simulink model "Distribution"  (R2015b)
settings: Solver=ode45  SolverMode=SingleTasking  StartTime=0.0  StopTime=500  RelTol=1e-3
libraries: simeventslib x10
(part 1 of 2)
settings Model: Creator=tsprock3  LastModifiedBy=tsprock3
settings DataIOCC: SaveFormat=Array
settings OptimizationCC: BlockReduction=off  BooleanDataType=off
settings DebuggingCC: SaveWithParameterizedLinksMsg=none  UnderspecifiedInitializationDetection=Classic  MergeDetectMultiDrivingBlocksExec=none  SignalResolutionControl=TryResolveAllWithWarning
settings HardwareCC: ProdBitPerPointer=32  ProdLargestAtomicFloat=None  ProdIntDivRoundTo=Undefined  ProdEndianess=Unspecified  ProdWordSize=32  ProdHWDeviceType=32-bit Generic  TargetUnknown=on
settings GRTTargetCC: GeneratePreprocessorConditionals=Disable all
settings ConfigComp: CovModelRefEnable=Off
settings SimEventsCC: propMaxDesBlkSimulEvents=100000  propMaxDesMdlSimulEvents=1000000

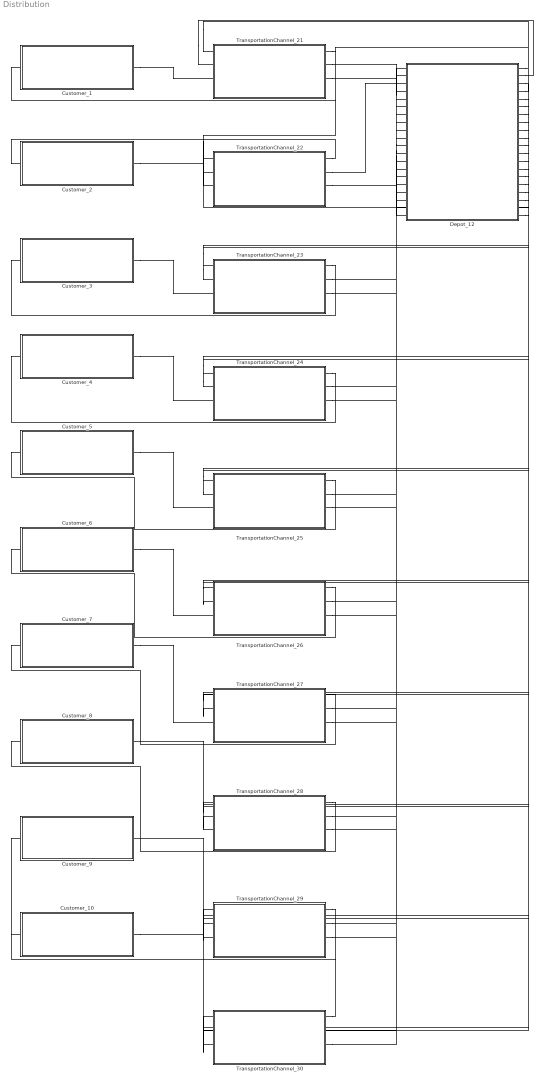
== system Distribution ==
  Customer_1 : Subsystem
  Customer_10 : Subsystem
  Customer_2 : Subsystem
  Customer_3 : Subsystem
  Customer_4 : Subsystem
  Customer_5 : Subsystem
  Customer_6 : Subsystem
  Customer_7 : Subsystem
  Customer_8 : Subsystem
  Customer_9 : Subsystem
  Depot_12 : Subsystem
  TransportationChannel_21 : Subsystem
  TransportationChannel_22 : Subsystem
  TransportationChannel_23 : Subsystem
  TransportationChannel_24 : Subsystem
  TransportationChannel_25 : Subsystem
  TransportationChannel_26 : Subsystem
  TransportationChannel_27 : Subsystem
  TransportationChannel_28 : Subsystem
  TransportationChannel_29 : Subsystem
  TransportationChannel_30 : Subsystem
  connections:
  Depot_12/RConn1 -- TransportationChannel_21/LConn1
  TransportationChannel_21/RConn1 -- Customer_1/LConn1
  Depot_12/RConn2 -- TransportationChannel_21/LConn2
  TransportationChannel_21/RConn2 -- Depot_12/LConn1
  Customer_1/RConn1 -- TransportationChannel_21/LConn3
  TransportationChannel_21/RConn3 -- Depot_12/LConn2
  Depot_12/RConn3 -- TransportationChannel_22/LConn1
  TransportationChannel_22/RConn1 -- Customer_2/LConn1
  Depot_12/RConn4 -- TransportationChannel_22/LConn2
  TransportationChannel_22/RConn2 -- Depot_12/LConn3
  Customer_2/RConn1 -- TransportationChannel_22/LConn3
  TransportationChannel_22/RConn3 -- Depot_12/LConn4
  Depot_12/RConn5 -- TransportationChannel_23/LConn1
  TransportationChannel_23/RConn1 -- Customer_3/LConn1
  Depot_12/RConn6 -- TransportationChannel_23/LConn2
  TransportationChannel_23/RConn2 -- Depot_12/LConn5
  Customer_3/RConn1 -- TransportationChannel_23/LConn3
  TransportationChannel_23/RConn3 -- Depot_12/LConn6
  Depot_12/RConn7 -- TransportationChannel_24/LConn1
  TransportationChannel_24/RConn1 -- Customer_4/LConn1
  Depot_12/RConn8 -- TransportationChannel_24/LConn2
  TransportationChannel_24/RConn2 -- Depot_12/LConn7
  Customer_4/RConn1 -- TransportationChannel_24/LConn3
  TransportationChannel_24/RConn3 -- Depot_12/LConn8
  Depot_12/RConn9 -- TransportationChannel_25/LConn1
  TransportationChannel_25/RConn1 -- Customer_5/LConn1
  Depot_12/RConn10 -- TransportationChannel_25/LConn2
  TransportationChannel_25/RConn2 -- Depot_12/LConn9
  Customer_5/RConn1 -- TransportationChannel_25/LConn3
  TransportationChannel_25/RConn3 -- Depot_12/LConn10
  Depot_12/RConn11 -- TransportationChannel_26/LConn1
  TransportationChannel_26/RConn1 -- Customer_6/LConn1
  Depot_12/RConn12 -- TransportationChannel_26/LConn2
  TransportationChannel_26/RConn2 -- Depot_12/LConn11
  Customer_6/RConn1 -- TransportationChannel_26/LConn3
  TransportationChannel_26/RConn3 -- Depot_12/LConn12
  Depot_12/RConn13 -- TransportationChannel_27/LConn1
  TransportationChannel_27/RConn1 -- Customer_7/LConn1
  Depot_12/RConn14 -- TransportationChannel_27/LConn2
  TransportationChannel_27/RConn2 -- Depot_12/LConn13
  Customer_7/RConn1 -- TransportationChannel_27/LConn3
  TransportationChannel_27/RConn3 -- Depot_12/LConn14
  Depot_12/RConn15 -- TransportationChannel_28/LConn1
  TransportationChannel_28/RConn1 -- Customer_8/LConn1
  Depot_12/RConn16 -- TransportationChannel_28/LConn2
  TransportationChannel_28/RConn2 -- Depot_12/LConn15
  Customer_8/RConn1 -- TransportationChannel_28/LConn3
  TransportationChannel_28/RConn3 -- Depot_12/LConn16
  Depot_12/RConn17 -- TransportationChannel_29/LConn1
  TransportationChannel_29/RConn1 -- Customer_9/LConn1
  Depot_12/RConn18 -- TransportationChannel_29/LConn2
  TransportationChannel_29/RConn2 -- Depot_12/LConn17
  Customer_9/RConn1 -- TransportationChannel_29/LConn3
  TransportationChannel_29/RConn3 -- Depot_12/LConn18
  Depot_12/RConn19 -- TransportationChannel_30/LConn1
  TransportationChannel_30/RConn1 -- Customer_10/LConn1
  Depot_12/RConn20 -- TransportationChannel_30/LConn2
  TransportationChannel_30/RConn2 -- Depot_12/LConn19
  Customer_10/RConn1 -- TransportationChannel_30/LConn3
  TransportationChannel_30/RConn3 -- Depot_12/LConn20

== system Distribution/Customer_1 ==
  Commodity_1 : Subsystem  mask{Mean=2000/2134, AttributeValue=[0]|1|0|1}
      mask prompts: Mean "Frequency"; AttributeValue "Attributes"
      mask TypeOptions Mean: Source/Mean
      mask TypeOptions AttributeValue: setAttribute/AttributeValue
  Entity Sink : EntitySink
  Get Attribute : GetAttribute  AttributeName=Origin|Destination|Start  AttributeMissing=Error|Error|Error  AttributeDefaultValue=1|1|1  AttributeTreatAsVector=1|1|1  AttributeSendTiming=After entity departure|After entity departure|After entity departure  EvaluatedDefaultAttributeValue={[];[];[]}
      settings: OutputPortMap=o1,o2,o3
  IN_Commodity : PathCombiner  NumberInputPorts=1
  IN_Shipment : PathCombiner  NumberInputPorts=1
  Mux : Mux  Inputs=3
  OUT_Shipment : OutputSwitch  NumberOutputPorts=1  SwitchingCriterion=From signal port p  AttributeName=Customer  StatNumberDeparted=on
  Routing : EventBasedRandomNumber  Distribution=Arbitrary discrete  valueVecDisc=[0,1]  probVecDisc=[0,1]  Seed=56944
  Shipment_Metrics : simeventslib/SimEvents Sinks/Discrete Event Signal to Workspace  VariableName=Customer_1  SaveFormat=Structure With Time  isMonitorOnly=off  isRecordIC=off
  Signal Latch : SignalLatch  InitialMemoryValue=1  ReadMemoryUpon=Write to memory event
      settings: InputPortMap=u0,u2  OutputPortMap=o2
  IN_Shipment_1 : PMIOPort  Port=1  Side=Left
  OUT_Shipment_1 : PMIOPort  Port=2  Side=Right
  wires:
  Signal Latch/1 -> OUT_Shipment/1
  OUT_Shipment/1 -> Signal Latch/1
  Routing/1 -> Signal Latch/2
  Mux/1 -> Shipment_Metrics/1
  Get Attribute/3 -> Mux/3
  Get Attribute/2 -> Mux/2
  Get Attribute/1 -> Mux/1
  connections:
  IN_Commodity/RConn1 -- OUT_Shipment/LConn1
  Get Attribute/LConn1 -- IN_Shipment/RConn1
  Entity Sink/LConn1 -- Get Attribute/RConn1
  IN_Shipment/LConn1 -- IN_Shipment_1/RConn1
  OUT_Shipment/RConn1 -- OUT_Shipment_1/RConn1
  Commodity_1/RConn1 -- IN_Commodity/LConn1

== system Distribution/Customer_10 ==
  Commodity_10 : Subsystem  mask{Mean=2000/1539, AttributeValue=[0]|10|0|1}
      mask prompts: Mean "Frequency"; AttributeValue "Attributes"
      mask TypeOptions Mean: Source/Mean
      mask TypeOptions AttributeValue: setAttribute/AttributeValue
  Entity Sink : EntitySink
  Get Attribute : GetAttribute  AttributeName=Origin|Destination|Start  AttributeMissing=Error|Error|Error  AttributeDefaultValue=1|1|1  AttributeTreatAsVector=1|1|1  AttributeSendTiming=After entity departure|After entity departure|After entity departure  EvaluatedDefaultAttributeValue={[];[];[]}
      settings: OutputPortMap=o1,o2,o3
  IN_Commodity : PathCombiner  NumberInputPorts=1
  IN_Shipment : PathCombiner  NumberInputPorts=1
  Mux : Mux  Inputs=3
  OUT_Shipment : OutputSwitch  NumberOutputPorts=1  SwitchingCriterion=From signal port p  AttributeName=Customer  StatNumberDeparted=on
  Routing : EventBasedRandomNumber  Distribution=Arbitrary discrete  valueVecDisc=[0,1]  probVecDisc=[0,1]  Seed=60161
  Shipment_Metrics : simeventslib/SimEvents Sinks/Discrete Event Signal to Workspace  VariableName=Customer_10  SaveFormat=Structure With Time  isMonitorOnly=off  isRecordIC=off
  Signal Latch : SignalLatch  InitialMemoryValue=1  ReadMemoryUpon=Write to memory event
      settings: InputPortMap=u0,u2  OutputPortMap=o2
  IN_Shipment_1 : PMIOPort  Port=1  Side=Left
  OUT_Shipment_1 : PMIOPort  Port=2  Side=Right
  wires:
  Signal Latch/1 -> OUT_Shipment/1
  OUT_Shipment/1 -> Signal Latch/1
  Routing/1 -> Signal Latch/2
  Mux/1 -> Shipment_Metrics/1
  Get Attribute/3 -> Mux/3
  Get Attribute/2 -> Mux/2
  Get Attribute/1 -> Mux/1
  connections:
  IN_Commodity/RConn1 -- OUT_Shipment/LConn1
  Get Attribute/LConn1 -- IN_Shipment/RConn1
  Entity Sink/LConn1 -- Get Attribute/RConn1
  IN_Shipment/LConn1 -- IN_Shipment_1/RConn1
  OUT_Shipment/RConn1 -- OUT_Shipment_1/RConn1
  Commodity_10/RConn1 -- IN_Commodity/LConn1

== system Distribution/Customer_2 ==
  Commodity_2 : Subsystem  mask{Mean=2000/1918, AttributeValue=[0]|2|0|1}
      mask prompts: Mean "Frequency"; AttributeValue "Attributes"
      mask TypeOptions Mean: Source/Mean
      mask TypeOptions AttributeValue: setAttribute/AttributeValue
  Entity Sink : EntitySink
  Get Attribute : GetAttribute  AttributeName=Origin|Destination|Start  AttributeMissing=Error|Error|Error  AttributeDefaultValue=1|1|1  AttributeTreatAsVector=1|1|1  AttributeSendTiming=After entity departure|After entity departure|After entity departure  EvaluatedDefaultAttributeValue={[];[];[]}
      settings: OutputPortMap=o1,o2,o3
  IN_Commodity : PathCombiner  NumberInputPorts=1
  IN_Shipment : PathCombiner  NumberInputPorts=1
  Mux : Mux  Inputs=3
  OUT_Shipment : OutputSwitch  NumberOutputPorts=1  SwitchingCriterion=From signal port p  AttributeName=Customer  StatNumberDeparted=on
  Routing : EventBasedRandomNumber  Distribution=Arbitrary discrete  valueVecDisc=[0,1]  probVecDisc=[0,1]  Seed=63378
  Shipment_Metrics : simeventslib/SimEvents Sinks/Discrete Event Signal to Workspace  VariableName=Customer_2  SaveFormat=Structure With Time  isMonitorOnly=off  isRecordIC=off
  Signal Latch : SignalLatch  InitialMemoryValue=1  ReadMemoryUpon=Write to memory event
      settings: InputPortMap=u0,u2  OutputPortMap=o2
  IN_Shipment_1 : PMIOPort  Port=1  Side=Left
  OUT_Shipment_1 : PMIOPort  Port=2  Side=Right
  wires:
  Signal Latch/1 -> OUT_Shipment/1
  OUT_Shipment/1 -> Signal Latch/1
  Routing/1 -> Signal Latch/2
  Mux/1 -> Shipment_Metrics/1
  Get Attribute/3 -> Mux/3
  Get Attribute/2 -> Mux/2
  Get Attribute/1 -> Mux/1
  connections:
  IN_Commodity/RConn1 -- OUT_Shipment/LConn1
  Get Attribute/LConn1 -- IN_Shipment/RConn1
  Entity Sink/LConn1 -- Get Attribute/RConn1
  IN_Shipment/LConn1 -- IN_Shipment_1/RConn1
  OUT_Shipment/RConn1 -- OUT_Shipment_1/RConn1
  Commodity_2/RConn1 -- IN_Commodity/LConn1

== system Distribution/Customer_3 ==
  Commodity_3 : Subsystem  mask{Mean=2000/1442, AttributeValue=[0]|3|0|1}
      mask prompts: Mean "Frequency"; AttributeValue "Attributes"
      mask TypeOptions Mean: Source/Mean
      mask TypeOptions AttributeValue: setAttribute/AttributeValue
  Entity Sink : EntitySink
  Get Attribute : GetAttribute  AttributeName=Origin|Destination|Start  AttributeMissing=Error|Error|Error  AttributeDefaultValue=1|1|1  AttributeTreatAsVector=1|1|1  AttributeSendTiming=After entity departure|After entity departure|After entity departure  EvaluatedDefaultAttributeValue={[];[];[]}
      settings: OutputPortMap=o1,o2,o3
  IN_Commodity : PathCombiner  NumberInputPorts=1
  IN_Shipment : PathCombiner  NumberInputPorts=1
  Mux : Mux  Inputs=3
  OUT_Shipment : OutputSwitch  NumberOutputPorts=1  SwitchingCriterion=From signal port p  AttributeName=Customer  StatNumberDeparted=on
  Routing : EventBasedRandomNumber  Distribution=Arbitrary discrete  valueVecDisc=[0,1]  probVecDisc=[0,1]  Seed=1059
  Shipment_Metrics : simeventslib/SimEvents Sinks/Discrete Event Signal to Workspace  VariableName=Customer_3  SaveFormat=Structure With Time  isMonitorOnly=off  isRecordIC=off
  Signal Latch : SignalLatch  InitialMemoryValue=1  ReadMemoryUpon=Write to memory event
      settings: InputPortMap=u0,u2  OutputPortMap=o2
  IN_Shipment_1 : PMIOPort  Port=1  Side=Left
  OUT_Shipment_1 : PMIOPort  Port=2  Side=Right
  wires:
  Signal Latch/1 -> OUT_Shipment/1
  OUT_Shipment/1 -> Signal Latch/1
  Routing/1 -> Signal Latch/2
  Mux/1 -> Shipment_Metrics/1
  Get Attribute/3 -> Mux/3
  Get Attribute/2 -> Mux/2
  Get Attribute/1 -> Mux/1
  connections:
  IN_Commodity/RConn1 -- OUT_Shipment/LConn1
  Get Attribute/LConn1 -- IN_Shipment/RConn1
  Entity Sink/LConn1 -- Get Attribute/RConn1
  IN_Shipment/LConn1 -- IN_Shipment_1/RConn1
  OUT_Shipment/RConn1 -- OUT_Shipment_1/RConn1
  Commodity_3/RConn1 -- IN_Commodity/LConn1

== system Distribution/Customer_4 ==
  Commodity_4 : Subsystem  mask{Mean=2000/1634, AttributeValue=[0]|4|0|1}
      mask prompts: Mean "Frequency"; AttributeValue "Attributes"
      mask TypeOptions Mean: Source/Mean
      mask TypeOptions AttributeValue: setAttribute/AttributeValue
  Entity Sink : EntitySink
  Get Attribute : GetAttribute  AttributeName=Origin|Destination|Start  AttributeMissing=Error|Error|Error  AttributeDefaultValue=1|1|1  AttributeTreatAsVector=1|1|1  AttributeSendTiming=After entity departure|After entity departure|After entity departure  EvaluatedDefaultAttributeValue={[];[];[]}
      settings: OutputPortMap=o1,o2,o3
  IN_Commodity : PathCombiner  NumberInputPorts=1
  IN_Shipment : PathCombiner  NumberInputPorts=1
  Mux : Mux  Inputs=3
  OUT_Shipment : OutputSwitch  NumberOutputPorts=1  SwitchingCriterion=From signal port p  AttributeName=Customer  StatNumberDeparted=on
  Routing : EventBasedRandomNumber  Distribution=Arbitrary discrete  valueVecDisc=[0,1]  probVecDisc=[0,1]  Seed=4276
  Shipment_Metrics : simeventslib/SimEvents Sinks/Discrete Event Signal to Workspace  VariableName=Customer_4  SaveFormat=Structure With Time  isMonitorOnly=off  isRecordIC=off
  Signal Latch : SignalLatch  InitialMemoryValue=1  ReadMemoryUpon=Write to memory event
      settings: InputPortMap=u0,u2  OutputPortMap=o2
  IN_Shipment_1 : PMIOPort  Port=1  Side=Left
  OUT_Shipment_1 : PMIOPort  Port=2  Side=Right
  wires:
  Signal Latch/1 -> OUT_Shipment/1
  OUT_Shipment/1 -> Signal Latch/1
  Routing/1 -> Signal Latch/2
  Mux/1 -> Shipment_Metrics/1
  Get Attribute/3 -> Mux/3
  Get Attribute/2 -> Mux/2
  Get Attribute/1 -> Mux/1
  connections:
  IN_Commodity/RConn1 -- OUT_Shipment/LConn1
  Get Attribute/LConn1 -- IN_Shipment/RConn1
  Entity Sink/LConn1 -- Get Attribute/RConn1
  IN_Shipment/LConn1 -- IN_Shipment_1/RConn1
  OUT_Shipment/RConn1 -- OUT_Shipment_1/RConn1
  Commodity_4/RConn1 -- IN_Commodity/LConn1

== system Distribution/Customer_5 ==
  Commodity_5 : Subsystem  mask{Mean=2000/1690, AttributeValue=[0]|5|0|1}
      mask prompts: Mean "Frequency"; AttributeValue "Attributes"
      mask TypeOptions Mean: Source/Mean
      mask TypeOptions AttributeValue: setAttribute/AttributeValue
  Entity Sink : EntitySink
  Get Attribute : GetAttribute  AttributeName=Origin|Destination|Start  AttributeMissing=Error|Error|Error  AttributeDefaultValue=1|1|1  AttributeTreatAsVector=1|1|1  AttributeSendTiming=After entity departure|After entity departure|After entity departure  EvaluatedDefaultAttributeValue={[];[];[]}
      settings: OutputPortMap=o1,o2,o3
  IN_Commodity : PathCombiner  NumberInputPorts=1
  IN_Shipment : PathCombiner  NumberInputPorts=1
  Mux : Mux  Inputs=3
  OUT_Shipment : OutputSwitch  NumberOutputPorts=1  SwitchingCriterion=From signal port p  AttributeName=Customer  StatNumberDeparted=on
  Routing : EventBasedRandomNumber  Distribution=Arbitrary discrete  valueVecDisc=[0,1]  probVecDisc=[0,1]  Seed=7493
  Shipment_Metrics : simeventslib/SimEvents Sinks/Discrete Event Signal to Workspace  VariableName=Customer_5  SaveFormat=Structure With Time  isMonitorOnly=off  isRecordIC=off
  Signal Latch : SignalLatch  InitialMemoryValue=1  ReadMemoryUpon=Write to memory event
      settings: InputPortMap=u0,u2  OutputPortMap=o2
  IN_Shipment_1 : PMIOPort  Port=1  Side=Left
  OUT_Shipment_1 : PMIOPort  Port=2  Side=Right
  wires:
  Signal Latch/1 -> OUT_Shipment/1
  OUT_Shipment/1 -> Signal Latch/1
  Routing/1 -> Signal Latch/2
  Mux/1 -> Shipment_Metrics/1
  Get Attribute/3 -> Mux/3
  Get Attribute/2 -> Mux/2
  Get Attribute/1 -> Mux/1
  connections:
  IN_Commodity/RConn1 -- OUT_Shipment/LConn1
  Get Attribute/LConn1 -- IN_Shipment/RConn1
  Entity Sink/LConn1 -- Get Attribute/RConn1
  IN_Shipment/LConn1 -- IN_Shipment_1/RConn1
  OUT_Shipment/RConn1 -- OUT_Shipment_1/RConn1
  Commodity_5/RConn1 -- IN_Commodity/LConn1

== system Distribution/Customer_6 ==
  Commodity_6 : Subsystem  mask{Mean=2000/1449, AttributeValue=[0]|6|0|1}
      mask prompts: Mean "Frequency"; AttributeValue "Attributes"
      mask TypeOptions Mean: Source/Mean
      mask TypeOptions AttributeValue: setAttribute/AttributeValue
  Entity Sink : EntitySink
  Get Attribute : GetAttribute  AttributeName=Origin|Destination|Start  AttributeMissing=Error|Error|Error  AttributeDefaultValue=1|1|1  AttributeTreatAsVector=1|1|1  AttributeSendTiming=After entity departure|After entity departure|After entity departure  EvaluatedDefaultAttributeValue={[];[];[]}
      settings: OutputPortMap=o1,o2,o3
  IN_Commodity : PathCombiner  NumberInputPorts=1
  IN_Shipment : PathCombiner  NumberInputPorts=1
  Mux : Mux  Inputs=3
  OUT_Shipment : OutputSwitch  NumberOutputPorts=1  SwitchingCriterion=From signal port p  AttributeName=Customer  StatNumberDeparted=on
  Routing : EventBasedRandomNumber  Distribution=Arbitrary discrete  valueVecDisc=[0,1]  probVecDisc=[0,1]  Seed=10710
  Shipment_Metrics : simeventslib/SimEvents Sinks/Discrete Event Signal to Workspace  VariableName=Customer_6  SaveFormat=Structure With Time  isMonitorOnly=off  isRecordIC=off
  Signal Latch : SignalLatch  InitialMemoryValue=1  ReadMemoryUpon=Write to memory event
      settings: InputPortMap=u0,u2  OutputPortMap=o2
  IN_Shipment_1 : PMIOPort  Port=1  Side=Left
  OUT_Shipment_1 : PMIOPort  Port=2  Side=Right
  wires:
  Signal Latch/1 -> OUT_Shipment/1
  OUT_Shipment/1 -> Signal Latch/1
  Routing/1 -> Signal Latch/2
  Mux/1 -> Shipment_Metrics/1
  Get Attribute/3 -> Mux/3
  Get Attribute/2 -> Mux/2
  Get Attribute/1 -> Mux/1
  connections:
  IN_Commodity/RConn1 -- OUT_Shipment/LConn1
  Get Attribute/LConn1 -- IN_Shipment/RConn1
  Entity Sink/LConn1 -- Get Attribute/RConn1
  IN_Shipment/LConn1 -- IN_Shipment_1/RConn1
  OUT_Shipment/RConn1 -- OUT_Shipment_1/RConn1
  Commodity_6/RConn1 -- IN_Commodity/LConn1

== system Distribution/Customer_7 ==
  Commodity_7 : Subsystem  mask{Mean=2000/1918, AttributeValue=[0]|7|0|1}
      mask prompts: Mean "Frequency"; AttributeValue "Attributes"
      mask TypeOptions Mean: Source/Mean
      mask TypeOptions AttributeValue: setAttribute/AttributeValue
  Entity Sink : EntitySink
  Get Attribute : GetAttribute  AttributeName=Origin|Destination|Start  AttributeMissing=Error|Error|Error  AttributeDefaultValue=1|1|1  AttributeTreatAsVector=1|1|1  AttributeSendTiming=After entity departure|After entity departure|After entity departure  EvaluatedDefaultAttributeValue={[];[];[]}
      settings: OutputPortMap=o1,o2,o3
  IN_Commodity : PathCombiner  NumberInputPorts=1
  IN_Shipment : PathCombiner  NumberInputPorts=1
  Mux : Mux  Inputs=3
  OUT_Shipment : OutputSwitch  NumberOutputPorts=1  SwitchingCriterion=From signal port p  AttributeName=Customer  StatNumberDeparted=on
  Routing : EventBasedRandomNumber  Distribution=Arbitrary discrete  valueVecDisc=[0,1]  probVecDisc=[0,1]  Seed=13927
  Shipment_Metrics : simeventslib/SimEvents Sinks/Discrete Event Signal to Workspace  VariableName=Customer_7  SaveFormat=Structure With Time  isMonitorOnly=off  isRecordIC=off
  Signal Latch : SignalLatch  InitialMemoryValue=1  ReadMemoryUpon=Write to memory event
      settings: InputPortMap=u0,u2  OutputPortMap=o2
  IN_Shipment_1 : PMIOPort  Port=1  Side=Left
  OUT_Shipment_1 : PMIOPort  Port=2  Side=Right
  wires:
  Signal Latch/1 -> OUT_Shipment/1
  OUT_Shipment/1 -> Signal Latch/1
  Routing/1 -> Signal Latch/2
  Mux/1 -> Shipment_Metrics/1
  Get Attribute/3 -> Mux/3
  Get Attribute/2 -> Mux/2
  Get Attribute/1 -> Mux/1
  connections:
  IN_Commodity/RConn1 -- OUT_Shipment/LConn1
  Get Attribute/LConn1 -- IN_Shipment/RConn1
  Entity Sink/LConn1 -- Get Attribute/RConn1
  IN_Shipment/LConn1 -- IN_Shipment_1/RConn1
  OUT_Shipment/RConn1 -- OUT_Shipment_1/RConn1
  Commodity_7/RConn1 -- IN_Commodity/LConn1

== system Distribution/Customer_8 ==
  Commodity_8 : Subsystem  mask{Mean=2000/1000, AttributeValue=[0]|8|0|1}
      mask prompts: Mean "Frequency"; AttributeValue "Attributes"
      mask TypeOptions Mean: Source/Mean
      mask TypeOptions AttributeValue: setAttribute/AttributeValue
  Entity Sink : EntitySink
  Get Attribute : GetAttribute  AttributeName=Origin|Destination|Start  AttributeMissing=Error|Error|Error  AttributeDefaultValue=1|1|1  AttributeTreatAsVector=1|1|1  AttributeSendTiming=After entity departure|After entity departure|After entity departure  EvaluatedDefaultAttributeValue={[];[];[]}
      settings: OutputPortMap=o1,o2,o3
  IN_Commodity : PathCombiner  NumberInputPorts=1
  IN_Shipment : PathCombiner  NumberInputPorts=1
  Mux : Mux  Inputs=3
  OUT_Shipment : OutputSwitch  NumberOutputPorts=1  SwitchingCriterion=From signal port p  AttributeName=Customer  StatNumberDeparted=on
  Routing : EventBasedRandomNumber  Distribution=Arbitrary discrete  valueVecDisc=[0,1]  probVecDisc=[0,1]  Seed=17144
  Shipment_Metrics : simeventslib/SimEvents Sinks/Discrete Event Signal to Workspace  VariableName=Customer_8  SaveFormat=Structure With Time  isMonitorOnly=off  isRecordIC=off
  Signal Latch : SignalLatch  InitialMemoryValue=1  ReadMemoryUpon=Write to memory event
      settings: InputPortMap=u0,u2  OutputPortMap=o2
  IN_Shipment_1 : PMIOPort  Port=1  Side=Left
  OUT_Shipment_1 : PMIOPort  Port=2  Side=Right
  wires:
  Signal Latch/1 -> OUT_Shipment/1
  OUT_Shipment/1 -> Signal Latch/1
  Routing/1 -> Signal Latch/2
  Mux/1 -> Shipment_Metrics/1
  Get Attribute/3 -> Mux/3
  Get Attribute/2 -> Mux/2
  Get Attribute/1 -> Mux/1
  connections:
  IN_Commodity/RConn1 -- OUT_Shipment/LConn1
  Get Attribute/LConn1 -- IN_Shipment/RConn1
  Entity Sink/LConn1 -- Get Attribute/RConn1
  IN_Shipment/LConn1 -- IN_Shipment_1/RConn1
  OUT_Shipment/RConn1 -- OUT_Shipment_1/RConn1
  Commodity_8/RConn1 -- IN_Commodity/LConn1

== system Distribution/Customer_9 ==
  Commodity_9 : Subsystem  mask{Mean=2000/2164, AttributeValue=[0]|9|0|1}
      mask prompts: Mean "Frequency"; AttributeValue "Attributes"
      mask TypeOptions Mean: Source/Mean
      mask TypeOptions AttributeValue: setAttribute/AttributeValue
  Entity Sink : EntitySink
  Get Attribute : GetAttribute  AttributeName=Origin|Destination|Start  AttributeMissing=Error|Error|Error  AttributeDefaultValue=1|1|1  AttributeTreatAsVector=1|1|1  AttributeSendTiming=After entity departure|After entity departure|After entity departure  EvaluatedDefaultAttributeValue={[];[];[]}
      settings: OutputPortMap=o1,o2,o3
  IN_Commodity : PathCombiner  NumberInputPorts=1
  IN_Shipment : PathCombiner  NumberInputPorts=1
  Mux : Mux  Inputs=3
  OUT_Shipment : OutputSwitch  NumberOutputPorts=1  SwitchingCriterion=From signal port p  AttributeName=Customer  StatNumberDeparted=on
  Routing : EventBasedRandomNumber  Distribution=Arbitrary discrete  valueVecDisc=[0,1]  probVecDisc=[0,1]  Seed=20361
  Shipment_Metrics : simeventslib/SimEvents Sinks/Discrete Event Signal to Workspace  VariableName=Customer_9  SaveFormat=Structure With Time  isMonitorOnly=off  isRecordIC=off
  Signal Latch : SignalLatch  InitialMemoryValue=1  ReadMemoryUpon=Write to memory event
      settings: InputPortMap=u0,u2  OutputPortMap=o2
  IN_Shipment_1 : PMIOPort  Port=1  Side=Left
  OUT_Shipment_1 : PMIOPort  Port=2  Side=Right
  wires:
  Signal Latch/1 -> OUT_Shipment/1
  OUT_Shipment/1 -> Signal Latch/1
  Routing/1 -> Signal Latch/2
  Mux/1 -> Shipment_Metrics/1
  Get Attribute/3 -> Mux/3
  Get Attribute/2 -> Mux/2
  Get Attribute/1 -> Mux/1
  connections:
  IN_Commodity/RConn1 -- OUT_Shipment/LConn1
  Get Attribute/LConn1 -- IN_Shipment/RConn1
  Entity Sink/LConn1 -- Get Attribute/RConn1
  IN_Shipment/LConn1 -- IN_Shipment_1/RConn1
  OUT_Shipment/RConn1 -- OUT_Shipment_1/RConn1
  Commodity_9/RConn1 -- IN_Commodity/LConn1

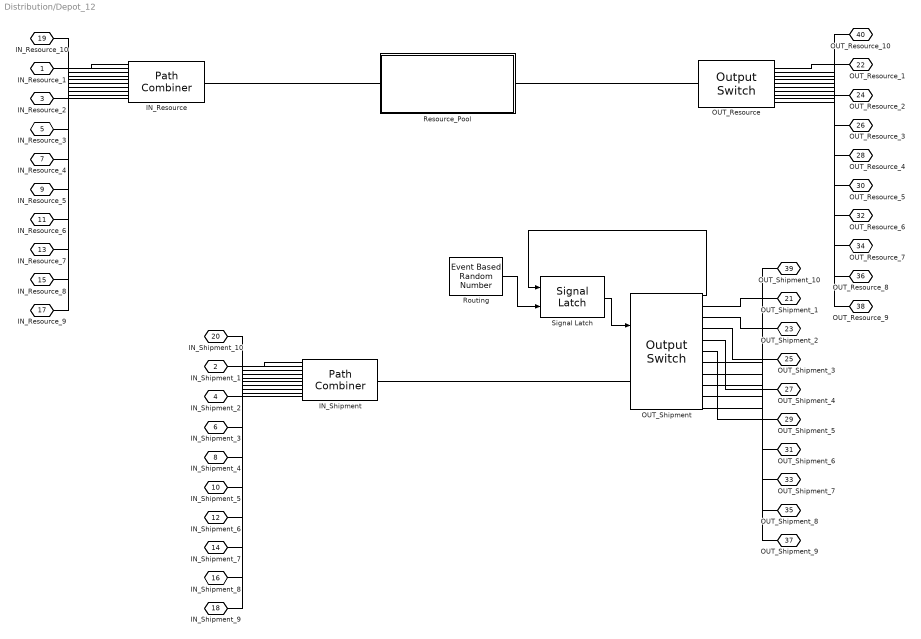
== system Distribution/Depot_12 ==
  IN_Resource : PathCombiner  NumberInputPorts=10
  IN_Shipment : PathCombiner  NumberInputPorts=10
  OUT_Resource : OutputSwitch  NumberOutputPorts=10  SwitchingCriterion=Round robin  InitialSeed=57769  StatLastDeparturePort=on
      settings: OutputPortMap=o3
  OUT_Shipment : OutputSwitch  NumberOutputPorts=10  SwitchingCriterion=From signal port p  AttributeName=Customer  StatNumberDeparted=on
  Resource_Pool : Subsystem  mask{Quantity=6}
      mask prompts: Quantity "How many entities in resource pool?"
      mask TypeOptions Quantity:
      | Time-Based
      | Function-Call Generator/NumberOfEventsPerPeriod
  Routing : EventBasedRandomNumber  Distribution=Arbitrary discrete  valueVecDisc=[0,1,2,3,4,5,6,7,8,9,10]  probVecDisc=[0,0.128,0.0796,0.0933,0.1586,0.1018,0.0731,0.1276,0.0545,0.0486,0.1349]  Seed=23578
  Signal Latch : SignalLatch  InitialMemoryValue=1  ReadMemoryUpon=Write to memory event
      settings: InputPortMap=u0,u2  OutputPortMap=o2
  IN_Resource_1 : PMIOPort  Port=1  Side=Left
  IN_Shipment_1 : PMIOPort  Port=2  Side=Left
  IN_Resource_2 : PMIOPort  Port=3  Side=Left
  IN_Shipment_2 : PMIOPort  Port=4  Side=Left
  IN_Resource_3 : PMIOPort  Port=5  Side=Left
  IN_Shipment_3 : PMIOPort  Port=6  Side=Left
  IN_Resource_4 : PMIOPort  Port=7  Side=Left
  IN_Shipment_4 : PMIOPort  Port=8  Side=Left
  IN_Resource_5 : PMIOPort  Port=9  Side=Left
  IN_Shipment_5 : PMIOPort  Port=10  Side=Left
  IN_Resource_6 : PMIOPort  Port=11  Side=Left
  IN_Shipment_6 : PMIOPort  Port=12  Side=Left
  IN_Resource_7 : PMIOPort  Port=13  Side=Left
  IN_Shipment_7 : PMIOPort  Port=14  Side=Left
  IN_Resource_8 : PMIOPort  Port=15  Side=Left
  IN_Shipment_8 : PMIOPort  Port=16  Side=Left
  IN_Resource_9 : PMIOPort  Port=17  Side=Left
  IN_Shipment_9 : PMIOPort  Port=18  Side=Left
  IN_Resource_10 : PMIOPort  Port=19  Side=Left
  IN_Shipment_10 : PMIOPort  Port=20  Side=Left
  OUT_Shipment_1 : PMIOPort  Port=21  Side=Right
  OUT_Resource_1 : PMIOPort  Port=22  Side=Right
  OUT_Shipment_2 : PMIOPort  Port=23  Side=Right
  OUT_Resource_2 : PMIOPort  Port=24  Side=Right
  OUT_Shipment_3 : PMIOPort  Port=25  Side=Right
  OUT_Resource_3 : PMIOPort  Port=26  Side=Right
  OUT_Shipment_4 : PMIOPort  Port=27  Side=Right
  OUT_Resource_4 : PMIOPort  Port=28  Side=Right
  OUT_Shipment_5 : PMIOPort  Port=29  Side=Right
  OUT_Resource_5 : PMIOPort  Port=30  Side=Right
  OUT_Shipment_6 : PMIOPort  Port=31  Side=Right
  OUT_Resource_6 : PMIOPort  Port=32  Side=Right
  OUT_Shipment_7 : PMIOPort  Port=33  Side=Right
  OUT_Resource_7 : PMIOPort  Port=34  Side=Right
  OUT_Shipment_8 : PMIOPort  Port=35  Side=Right
  OUT_Resource_8 : PMIOPort  Port=36  Side=Right
  OUT_Shipment_9 : PMIOPort  Port=37  Side=Right
  OUT_Resource_9 : PMIOPort  Port=38  Side=Right
  OUT_Shipment_10 : PMIOPort  Port=39  Side=Right
  OUT_Resource_10 : PMIOPort  Port=40  Side=Right
  wires:
  OUT_Shipment/1 -> Signal Latch/1
  Routing/1 -> Signal Latch/2
  Signal Latch/1 -> OUT_Shipment/1
  connections:
  Resource_Pool/LConn1 -- OUT_Resource/LConn1
  IN_Shipment/RConn1 -- OUT_Shipment/LConn1
  Resource_Pool/RConn1 -- IN_Resource/RConn1
  IN_Resource/LConn1 -- IN_Resource_1/RConn1
  IN_Resource/LConn2 -- IN_Resource_2/RConn1
  IN_Resource/LConn3 -- IN_Resource_3/RConn1
  IN_Resource/LConn4 -- IN_Resource_4/RConn1
  IN_Resource/LConn5 -- IN_Resource_5/RConn1
  IN_Resource/LConn6 -- IN_Resource_6/RConn1
  IN_Resource/LConn7 -- IN_Resource_7/RConn1
  IN_Resource/LConn8 -- IN_Resource_8/RConn1
  IN_Resource/LConn9 -- IN_Resource_9/RConn1
  IN_Resource/LConn10 -- IN_Resource_10/RConn1
  OUT_Resource/RConn1 -- OUT_Resource_1/RConn1
  OUT_Resource/RConn2 -- OUT_Resource_2/RConn1
  OUT_Resource/RConn3 -- OUT_Resource_3/RConn1
  OUT_Resource/RConn4 -- OUT_Resource_4/RConn1
  OUT_Resource/RConn5 -- OUT_Resource_5/RConn1
  OUT_Resource/RConn6 -- OUT_Resource_6/RConn1
  OUT_Resource/RConn7 -- OUT_Resource_7/RConn1
  OUT_Resource/RConn8 -- OUT_Resource_8/RConn1
  OUT_Resource/RConn9 -- OUT_Resource_9/RConn1
  OUT_Resource/RConn10 -- OUT_Resource_10/RConn1
  IN_Shipment/LConn1 -- IN_Shipment_1/RConn1
  IN_Shipment/LConn2 -- IN_Shipment_2/RConn1
  IN_Shipment/LConn3 -- IN_Shipment_3/RConn1
  IN_Shipment/LConn4 -- IN_Shipment_4/RConn1
  IN_Shipment/LConn5 -- IN_Shipment_5/RConn1
  IN_Shipment/LConn6 -- IN_Shipment_6/RConn1
  IN_Shipment/LConn7 -- IN_Shipment_7/RConn1
  IN_Shipment/LConn8 -- IN_Shipment_8/RConn1
  IN_Shipment/LConn9 -- IN_Shipment_9/RConn1
  IN_Shipment/LConn10 -- IN_Shipment_10/RConn1
  OUT_Shipment/RConn1 -- OUT_Shipment_1/RConn1
  OUT_Shipment/RConn2 -- OUT_Shipment_2/RConn1
  OUT_Shipment/RConn3 -- OUT_Shipment_3/RConn1
  OUT_Shipment/RConn4 -- OUT_Shipment_4/RConn1
  OUT_Shipment/RConn5 -- OUT_Shipment_5/RConn1
  OUT_Shipment/RConn6 -- OUT_Shipment_6/RConn1
  OUT_Shipment/RConn7 -- OUT_Shipment_7/RConn1
  OUT_Shipment/RConn8 -- OUT_Shipment_8/RConn1
  OUT_Shipment/RConn9 -- OUT_Shipment_9/RConn1
  OUT_Shipment/RConn10 -- OUT_Shipment_10/RConn1

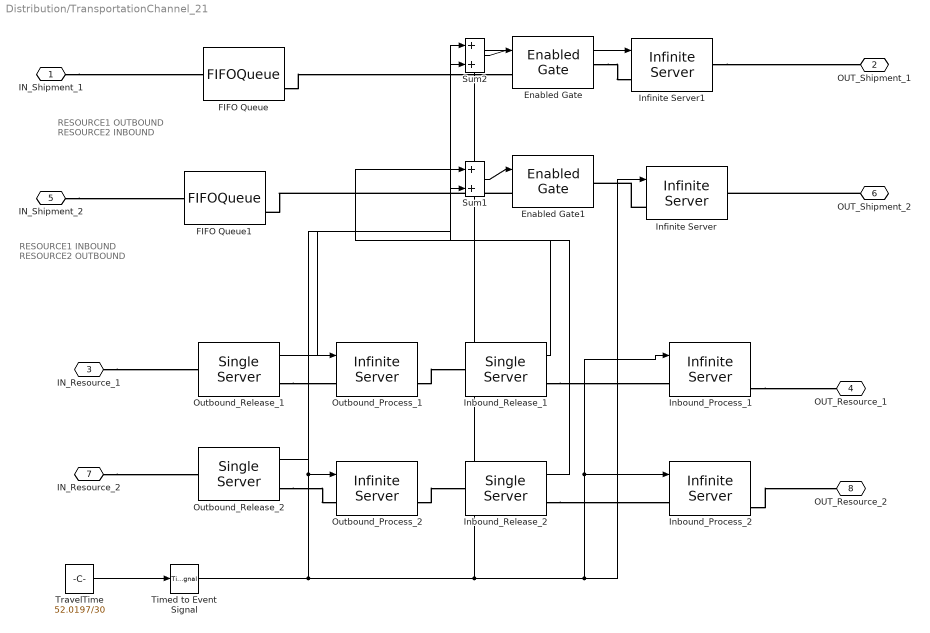
== system Distribution/TransportationChannel_21 ==
  note: RESOURCE1 OUTBOUND
      | RESOURCE2 INBOUND
  note: RESOURCE1 INBOUND
      | RESOURCE2 OUTBOUND
  Enabled Gate : EnabledGate
  Enabled Gate1 : EnabledGate
  FIFO Queue : FIFOQueue  Capacity=inf  StatNumberInBlock=on
      settings: OutputPortMap=o1
  FIFO Queue1 : FIFOQueue  Capacity=inf  StatNumberInBlock=on
      settings: OutputPortMap=o1
  Inbound_Process_1 : InfiniteServer  ServiceTimeFrom=Signal port t  ServiceTime=(76.7)/30  StatNumberDeparted=on  StatNumberInBlock=on
      settings: OutputPortMap=o0,o1
  Inbound_Process_2 : InfiniteServer  ServiceTimeFrom=Signal port t  ServiceTime=(76.7)/30  StatNumberDeparted=on  StatNumberInBlock=on
      settings: OutputPortMap=o0,o1
  Inbound_Release_1 : SingleServer  ServiceTime=0  StatNumberInBlock=on
      settings: OutputPortMap=o1
  Inbound_Release_2 : SingleServer  ServiceTime=0  StatNumberInBlock=on
      settings: OutputPortMap=o1
  Infinite Server : InfiniteServer  ServiceTimeFrom=Signal port t  ServiceTime=(76.7)/30
  Infinite Server1 : InfiniteServer  ServiceTimeFrom=Signal port t  ServiceTime=(76.7)/30
  Outbound_Process_1 : InfiniteServer  ServiceTimeFrom=Signal port t  ServiceTime=(76.7)/30  StatNumberInBlock=on
      settings: OutputPortMap=o1
  Outbound_Process_2 : InfiniteServer  ServiceTimeFrom=Signal port t  ServiceTime=(76.7)/30  StatNumberInBlock=on
      settings: OutputPortMap=o1
  Outbound_Release_1 : SingleServer  ServiceTime=0  StatNumberInBlock=on
      settings: OutputPortMap=o1
  Outbound_Release_2 : SingleServer  ServiceTime=0  StatNumberInBlock=on
      settings: OutputPortMap=o1
  Sum1 : Sum  Inputs=|++
  Sum2 : Sum  Inputs=|++
  Timed to Event Signal : TimedToEventSignal
  TravelTime : Constant  Value=52.0197/30
  IN_Shipment_1 : PMIOPort  Port=1  Side=Left
  OUT_Shipment_1 : PMIOPort  Port=2  Side=Right
  IN_Resource_1 : PMIOPort  Port=3  Side=Left
  OUT_Resource_1 : PMIOPort  Port=4  Side=Right
  IN_Shipment_2 : PMIOPort  Port=5  Side=Left
  OUT_Shipment_2 : PMIOPort  Port=6  Side=Right
  IN_Resource_2 : PMIOPort  Port=7  Side=Left
  OUT_Resource_2 : PMIOPort  Port=8  Side=Right
  wires:
  Inbound_Release_2/1 -> Sum2/2
  Outbound_Release_1/1 -> Sum2/1
  Sum2/1 -> Enabled Gate/1
  Inbound_Release_1/1 -> Sum1/1
  Outbound_Release_2/1 -> Sum1/2
  Sum1/1 -> Enabled Gate1/1
  Timed to Event Signal/1 -> Outbound_Process_2/1, Outbound_Process_1/1, Infinite Server1/1, Inbound_Process_2/1, Inbound_Process_1/1, Infinite Server/1
  TravelTime/1 -> Timed to Event Signal/1
  connections:
  Inbound_Process_1/RConn1 -- OUT_Resource_1/RConn1
  Outbound_Process_1/RConn1 -- Inbound_Release_1/LConn1
  Inbound_Release_1/RConn1 -- Inbound_Process_1/LConn1
  Outbound_Release_1/RConn1 -- Outbound_Process_1/LConn1
  Inbound_Process_2/RConn1 -- OUT_Resource_2/RConn1
  Inbound_Release_2/RConn1 -- Inbound_Process_2/LConn1
  Outbound_Process_2/RConn1 -- Inbound_Release_2/LConn1
  Outbound_Release_2/RConn1 -- Outbound_Process_2/LConn1
  IN_Resource_2/RConn1 -- Outbound_Release_2/LConn1
  Infinite Server1/RConn1 -- OUT_Shipment_1/RConn1
  Enabled Gate/RConn1 -- Infinite Server1/LConn1
  Infinite Server/LConn1 -- Enabled Gate1/RConn1
  OUT_Shipment_2/RConn1 -- Infinite Server/RConn1
  IN_Resource_1/RConn1 -- Outbound_Release_1/LConn1
  IN_Shipment_2/RConn1 -- FIFO Queue1/LConn1
  IN_Shipment_1/RConn1 -- FIFO Queue/LConn1
  Enabled Gate1/LConn1 -- FIFO Queue1/RConn1
  FIFO Queue/RConn1 -- Enabled Gate/LConn1

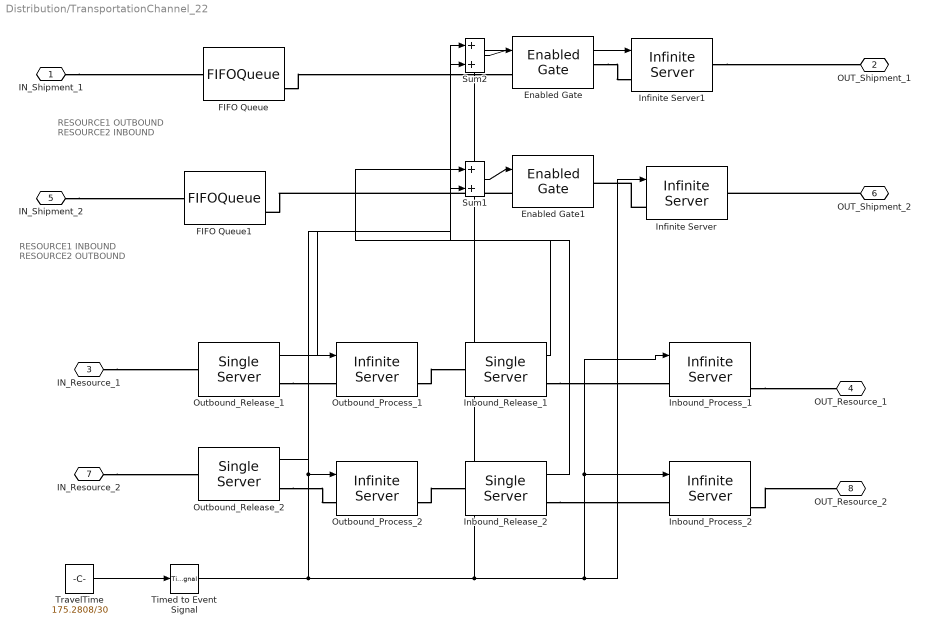
== system Distribution/TransportationChannel_22 ==
  note: RESOURCE1 OUTBOUND
      | RESOURCE2 INBOUND
  note: RESOURCE1 INBOUND
      | RESOURCE2 OUTBOUND
  Enabled Gate : EnabledGate
  Enabled Gate1 : EnabledGate
  FIFO Queue : FIFOQueue  Capacity=inf  StatNumberInBlock=on
      settings: OutputPortMap=o1
  FIFO Queue1 : FIFOQueue  Capacity=inf  StatNumberInBlock=on
      settings: OutputPortMap=o1
  Inbound_Process_1 : InfiniteServer  ServiceTimeFrom=Signal port t  ServiceTime=(76.7)/30  StatNumberDeparted=on  StatNumberInBlock=on
      settings: OutputPortMap=o0,o1
  Inbound_Process_2 : InfiniteServer  ServiceTimeFrom=Signal port t  ServiceTime=(76.7)/30  StatNumberDeparted=on  StatNumberInBlock=on
      settings: OutputPortMap=o0,o1
  Inbound_Release_1 : SingleServer  ServiceTime=0  StatNumberInBlock=on
      settings: OutputPortMap=o1
  Inbound_Release_2 : SingleServer  ServiceTime=0  StatNumberInBlock=on
      settings: OutputPortMap=o1
  Infinite Server : InfiniteServer  ServiceTimeFrom=Signal port t  ServiceTime=(76.7)/30
  Infinite Server1 : InfiniteServer  ServiceTimeFrom=Signal port t  ServiceTime=(76.7)/30
  Outbound_Process_1 : InfiniteServer  ServiceTimeFrom=Signal port t  ServiceTime=(76.7)/30  StatNumberInBlock=on
      settings: OutputPortMap=o1
  Outbound_Process_2 : InfiniteServer  ServiceTimeFrom=Signal port t  ServiceTime=(76.7)/30  StatNumberInBlock=on
      settings: OutputPortMap=o1
  Outbound_Release_1 : SingleServer  ServiceTime=0  StatNumberInBlock=on
      settings: OutputPortMap=o1
  Outbound_Release_2 : SingleServer  ServiceTime=0  StatNumberInBlock=on
      settings: OutputPortMap=o1
  Sum1 : Sum  Inputs=|++
  Sum2 : Sum  Inputs=|++
  Timed to Event Signal : TimedToEventSignal
  TravelTime : Constant  Value=175.2808/30
  IN_Shipment_1 : PMIOPort  Port=1  Side=Left
  OUT_Shipment_1 : PMIOPort  Port=2  Side=Right
  IN_Resource_1 : PMIOPort  Port=3  Side=Left
  OUT_Resource_1 : PMIOPort  Port=4  Side=Right
  IN_Shipment_2 : PMIOPort  Port=5  Side=Left
  OUT_Shipment_2 : PMIOPort  Port=6  Side=Right
  IN_Resource_2 : PMIOPort  Port=7  Side=Left
  OUT_Resource_2 : PMIOPort  Port=8  Side=Right
  wires:
  Inbound_Release_2/1 -> Sum2/2
  Outbound_Release_1/1 -> Sum2/1
  Sum2/1 -> Enabled Gate/1
  Inbound_Release_1/1 -> Sum1/1
  Outbound_Release_2/1 -> Sum1/2
  Sum1/1 -> Enabled Gate1/1
  Timed to Event Signal/1 -> Outbound_Process_2/1, Outbound_Process_1/1, Infinite Server1/1, Inbound_Process_2/1, Inbound_Process_1/1, Infinite Server/1
  TravelTime/1 -> Timed to Event Signal/1
  connections:
  Inbound_Process_1/RConn1 -- OUT_Resource_1/RConn1
  Outbound_Process_1/RConn1 -- Inbound_Release_1/LConn1
  Inbound_Release_1/RConn1 -- Inbound_Process_1/LConn1
  Outbound_Release_1/RConn1 -- Outbound_Process_1/LConn1
  Inbound_Process_2/RConn1 -- OUT_Resource_2/RConn1
  Inbound_Release_2/RConn1 -- Inbound_Process_2/LConn1
  Outbound_Process_2/RConn1 -- Inbound_Release_2/LConn1
  Outbound_Release_2/RConn1 -- Outbound_Process_2/LConn1
  IN_Resource_2/RConn1 -- Outbound_Release_2/LConn1
  Infinite Server1/RConn1 -- OUT_Shipment_1/RConn1
  Enabled Gate/RConn1 -- Infinite Server1/LConn1
  Infinite Server/LConn1 -- Enabled Gate1/RConn1
  OUT_Shipment_2/RConn1 -- Infinite Server/RConn1
  IN_Resource_1/RConn1 -- Outbound_Release_1/LConn1
  IN_Shipment_2/RConn1 -- FIFO Queue1/LConn1
  IN_Shipment_1/RConn1 -- FIFO Queue/LConn1
  Enabled Gate1/LConn1 -- FIFO Queue1/RConn1
  FIFO Queue/RConn1 -- Enabled Gate/LConn1

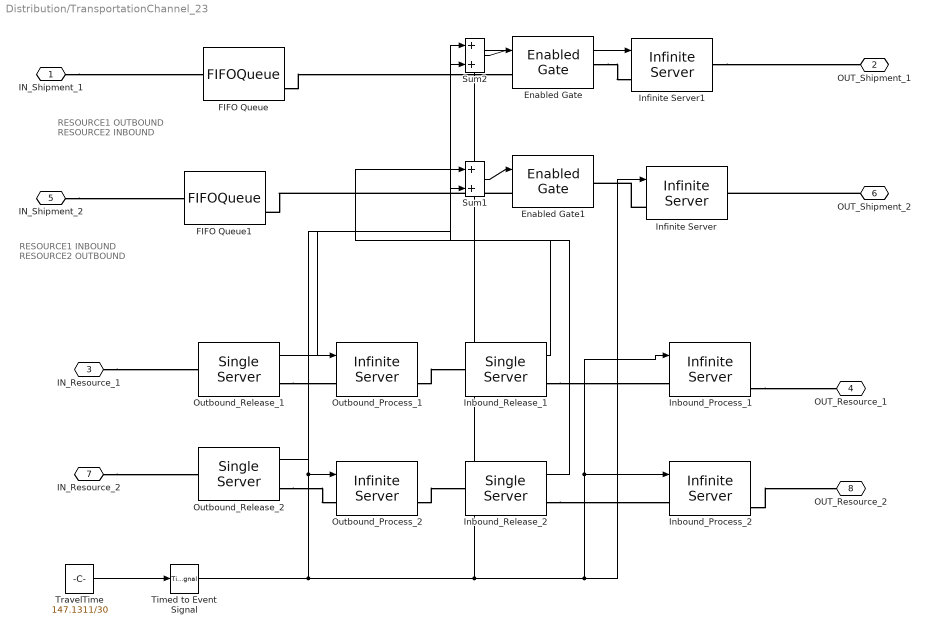
== system Distribution/TransportationChannel_23 ==
  note: RESOURCE1 OUTBOUND
      | RESOURCE2 INBOUND
  note: RESOURCE1 INBOUND
      | RESOURCE2 OUTBOUND
  Enabled Gate : EnabledGate
  Enabled Gate1 : EnabledGate
  FIFO Queue : FIFOQueue  Capacity=inf  StatNumberInBlock=on
      settings: OutputPortMap=o1
  FIFO Queue1 : FIFOQueue  Capacity=inf  StatNumberInBlock=on
      settings: OutputPortMap=o1
  Inbound_Process_1 : InfiniteServer  ServiceTimeFrom=Signal port t  ServiceTime=(76.7)/30  StatNumberDeparted=on  StatNumberInBlock=on
      settings: OutputPortMap=o0,o1
  Inbound_Process_2 : InfiniteServer  ServiceTimeFrom=Signal port t  ServiceTime=(76.7)/30  StatNumberDeparted=on  StatNumberInBlock=on
      settings: OutputPortMap=o0,o1
  Inbound_Release_1 : SingleServer  ServiceTime=0  StatNumberInBlock=on
      settings: OutputPortMap=o1
  Inbound_Release_2 : SingleServer  ServiceTime=0  StatNumberInBlock=on
      settings: OutputPortMap=o1
  Infinite Server : InfiniteServer  ServiceTimeFrom=Signal port t  ServiceTime=(76.7)/30
  Infinite Server1 : InfiniteServer  ServiceTimeFrom=Signal port t  ServiceTime=(76.7)/30
  Outbound_Process_1 : InfiniteServer  ServiceTimeFrom=Signal port t  ServiceTime=(76.7)/30  StatNumberInBlock=on
      settings: OutputPortMap=o1
  Outbound_Process_2 : InfiniteServer  ServiceTimeFrom=Signal port t  ServiceTime=(76.7)/30  StatNumberInBlock=on
      settings: OutputPortMap=o1
  Outbound_Release_1 : SingleServer  ServiceTime=0  StatNumberInBlock=on
      settings: OutputPortMap=o1
  Outbound_Release_2 : SingleServer  ServiceTime=0  StatNumberInBlock=on
      settings: OutputPortMap=o1
  Sum1 : Sum  Inputs=|++
  Sum2 : Sum  Inputs=|++
  Timed to Event Signal : TimedToEventSignal
  TravelTime : Constant  Value=147.1311/30
  IN_Shipment_1 : PMIOPort  Port=1  Side=Left
  OUT_Shipment_1 : PMIOPort  Port=2  Side=Right
  IN_Resource_1 : PMIOPort  Port=3  Side=Left
  OUT_Resource_1 : PMIOPort  Port=4  Side=Right
  IN_Shipment_2 : PMIOPort  Port=5  Side=Left
  OUT_Shipment_2 : PMIOPort  Port=6  Side=Right
  IN_Resource_2 : PMIOPort  Port=7  Side=Left
  OUT_Resource_2 : PMIOPort  Port=8  Side=Right
  wires:
  Inbound_Release_2/1 -> Sum2/2
  Outbound_Release_1/1 -> Sum2/1
  Sum2/1 -> Enabled Gate/1
  Inbound_Release_1/1 -> Sum1/1
  Outbound_Release_2/1 -> Sum1/2
  Sum1/1 -> Enabled Gate1/1
  Timed to Event Signal/1 -> Outbound_Process_2/1, Outbound_Process_1/1, Infinite Server1/1, Inbound_Process_2/1, Inbound_Process_1/1, Infinite Server/1
  TravelTime/1 -> Timed to Event Signal/1
  connections:
  Inbound_Process_1/RConn1 -- OUT_Resource_1/RConn1
  Outbound_Process_1/RConn1 -- Inbound_Release_1/LConn1
  Inbound_Release_1/RConn1 -- Inbound_Process_1/LConn1
  Outbound_Release_1/RConn1 -- Outbound_Process_1/LConn1
  Inbound_Process_2/RConn1 -- OUT_Resource_2/RConn1
  Inbound_Release_2/RConn1 -- Inbound_Process_2/LConn1
  Outbound_Process_2/RConn1 -- Inbound_Release_2/LConn1
  Outbound_Release_2/RConn1 -- Outbound_Process_2/LConn1
  IN_Resource_2/RConn1 -- Outbound_Release_2/LConn1
  Infinite Server1/RConn1 -- OUT_Shipment_1/RConn1
  Enabled Gate/RConn1 -- Infinite Server1/LConn1
  Infinite Server/LConn1 -- Enabled Gate1/RConn1
  OUT_Shipment_2/RConn1 -- Infinite Server/RConn1
  IN_Resource_1/RConn1 -- Outbound_Release_1/LConn1
  IN_Shipment_2/RConn1 -- FIFO Queue1/LConn1
  IN_Shipment_1/RConn1 -- FIFO Queue/LConn1
  Enabled Gate1/LConn1 -- FIFO Queue1/RConn1
  FIFO Queue/RConn1 -- Enabled Gate/LConn1

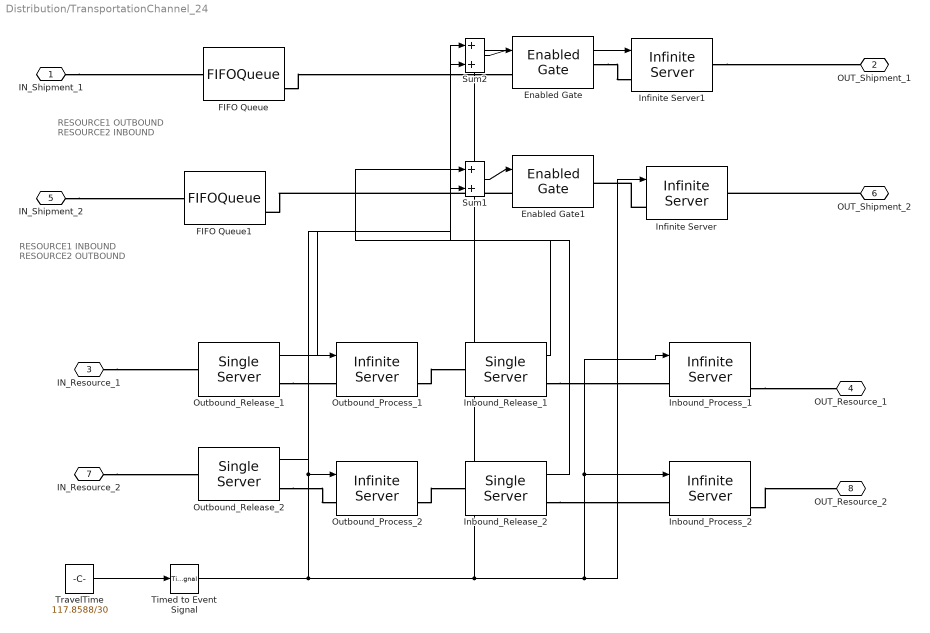
== system Distribution/TransportationChannel_24 ==
  note: RESOURCE1 OUTBOUND
      | RESOURCE2 INBOUND
  note: RESOURCE1 INBOUND
      | RESOURCE2 OUTBOUND
  Enabled Gate : EnabledGate
  Enabled Gate1 : EnabledGate
  FIFO Queue : FIFOQueue  Capacity=inf  StatNumberInBlock=on
      settings: OutputPortMap=o1
  FIFO Queue1 : FIFOQueue  Capacity=inf  StatNumberInBlock=on
      settings: OutputPortMap=o1
  Inbound_Process_1 : InfiniteServer  ServiceTimeFrom=Signal port t  ServiceTime=(76.7)/30  StatNumberDeparted=on  StatNumberInBlock=on
      settings: OutputPortMap=o0,o1
  Inbound_Process_2 : InfiniteServer  ServiceTimeFrom=Signal port t  ServiceTime=(76.7)/30  StatNumberDeparted=on  StatNumberInBlock=on
      settings: OutputPortMap=o0,o1
  Inbound_Release_1 : SingleServer  ServiceTime=0  StatNumberInBlock=on
      settings: OutputPortMap=o1
  Inbound_Release_2 : SingleServer  ServiceTime=0  StatNumberInBlock=on
      settings: OutputPortMap=o1
  Infinite Server : InfiniteServer  ServiceTimeFrom=Signal port t  ServiceTime=(76.7)/30
  Infinite Server1 : InfiniteServer  ServiceTimeFrom=Signal port t  ServiceTime=(76.7)/30
  Outbound_Process_1 : InfiniteServer  ServiceTimeFrom=Signal port t  ServiceTime=(76.7)/30  StatNumberInBlock=on
      settings: OutputPortMap=o1
  Outbound_Process_2 : InfiniteServer  ServiceTimeFrom=Signal port t  ServiceTime=(76.7)/30  StatNumberInBlock=on
      settings: OutputPortMap=o1
  Outbound_Release_1 : SingleServer  ServiceTime=0  StatNumberInBlock=on
      settings: OutputPortMap=o1
  Outbound_Release_2 : SingleServer  ServiceTime=0  StatNumberInBlock=on
      settings: OutputPortMap=o1
  Sum1 : Sum  Inputs=|++
  Sum2 : Sum  Inputs=|++
  Timed to Event Signal : TimedToEventSignal
  TravelTime : Constant  Value=117.8588/30
  IN_Shipment_1 : PMIOPort  Port=1  Side=Left
  OUT_Shipment_1 : PMIOPort  Port=2  Side=Right
  IN_Resource_1 : PMIOPort  Port=3  Side=Left
  OUT_Resource_1 : PMIOPort  Port=4  Side=Right
  IN_Shipment_2 : PMIOPort  Port=5  Side=Left
  OUT_Shipment_2 : PMIOPort  Port=6  Side=Right
  IN_Resource_2 : PMIOPort  Port=7  Side=Left
  OUT_Resource_2 : PMIOPort  Port=8  Side=Right
  wires:
  Inbound_Release_2/1 -> Sum2/2
  Outbound_Release_1/1 -> Sum2/1
  Sum2/1 -> Enabled Gate/1
  Inbound_Release_1/1 -> Sum1/1
  Outbound_Release_2/1 -> Sum1/2
  Sum1/1 -> Enabled Gate1/1
  Timed to Event Signal/1 -> Outbound_Process_2/1, Outbound_Process_1/1, Infinite Server1/1, Inbound_Process_2/1, Inbound_Process_1/1, Infinite Server/1
  TravelTime/1 -> Timed to Event Signal/1
  connections:
  Inbound_Process_1/RConn1 -- OUT_Resource_1/RConn1
  Outbound_Process_1/RConn1 -- Inbound_Release_1/LConn1
  Inbound_Release_1/RConn1 -- Inbound_Process_1/LConn1
  Outbound_Release_1/RConn1 -- Outbound_Process_1/LConn1
  Inbound_Process_2/RConn1 -- OUT_Resource_2/RConn1
  Inbound_Release_2/RConn1 -- Inbound_Process_2/LConn1
  Outbound_Process_2/RConn1 -- Inbound_Release_2/LConn1
  Outbound_Release_2/RConn1 -- Outbound_Process_2/LConn1
  IN_Resource_2/RConn1 -- Outbound_Release_2/LConn1
  Infinite Server1/RConn1 -- OUT_Shipment_1/RConn1
  Enabled Gate/RConn1 -- Infinite Server1/LConn1
  Infinite Server/LConn1 -- Enabled Gate1/RConn1
  OUT_Shipment_2/RConn1 -- Infinite Server/RConn1
  IN_Resource_1/RConn1 -- Outbound_Release_1/LConn1
  IN_Shipment_2/RConn1 -- FIFO Queue1/LConn1
  IN_Shipment_1/RConn1 -- FIFO Queue/LConn1
  Enabled Gate1/LConn1 -- FIFO Queue1/RConn1
  FIFO Queue/RConn1 -- Enabled Gate/LConn1

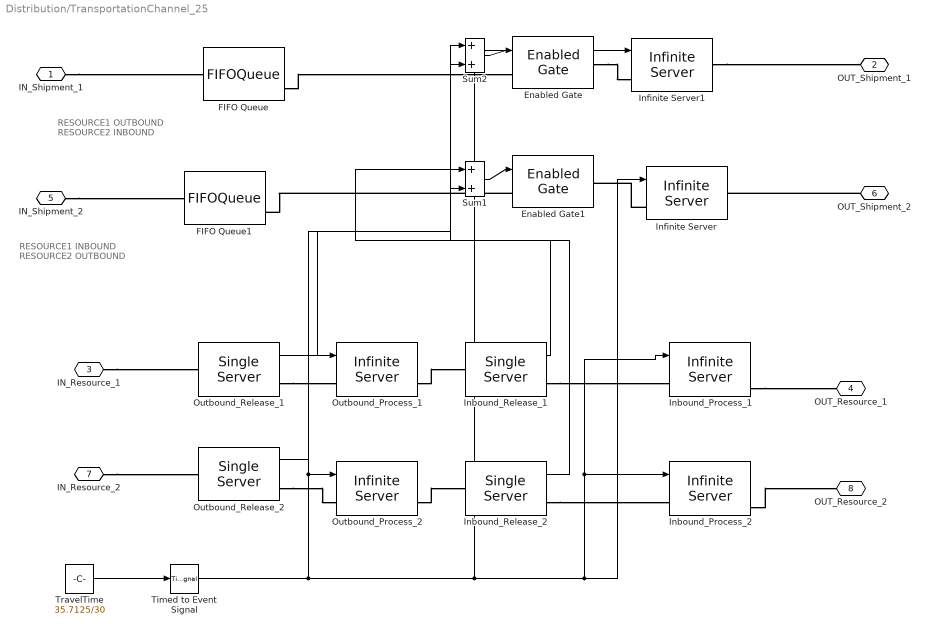
== system Distribution/TransportationChannel_25 ==
  note: RESOURCE1 OUTBOUND
      | RESOURCE2 INBOUND
  note: RESOURCE1 INBOUND
      | RESOURCE2 OUTBOUND
  Enabled Gate : EnabledGate
  Enabled Gate1 : EnabledGate
  FIFO Queue : FIFOQueue  Capacity=inf  StatNumberInBlock=on
      settings: OutputPortMap=o1
  FIFO Queue1 : FIFOQueue  Capacity=inf  StatNumberInBlock=on
      settings: OutputPortMap=o1
  Inbound_Process_1 : InfiniteServer  ServiceTimeFrom=Signal port t  ServiceTime=(76.7)/30  StatNumberDeparted=on  StatNumberInBlock=on
      settings: OutputPortMap=o0,o1
  Inbound_Process_2 : InfiniteServer  ServiceTimeFrom=Signal port t  ServiceTime=(76.7)/30  StatNumberDeparted=on  StatNumberInBlock=on
      settings: OutputPortMap=o0,o1
  Inbound_Release_1 : SingleServer  ServiceTime=0  StatNumberInBlock=on
      settings: OutputPortMap=o1
  Inbound_Release_2 : SingleServer  ServiceTime=0  StatNumberInBlock=on
      settings: OutputPortMap=o1
  Infinite Server : InfiniteServer  ServiceTimeFrom=Signal port t  ServiceTime=(76.7)/30
  Infinite Server1 : InfiniteServer  ServiceTimeFrom=Signal port t  ServiceTime=(76.7)/30
  Outbound_Process_1 : InfiniteServer  ServiceTimeFrom=Signal port t  ServiceTime=(76.7)/30  StatNumberInBlock=on
      settings: OutputPortMap=o1
  Outbound_Process_2 : InfiniteServer  ServiceTimeFrom=Signal port t  ServiceTime=(76.7)/30  StatNumberInBlock=on
      settings: OutputPortMap=o1
  Outbound_Release_1 : SingleServer  ServiceTime=0  StatNumberInBlock=on
      settings: OutputPortMap=o1
  Outbound_Release_2 : SingleServer  ServiceTime=0  StatNumberInBlock=on
      settings: OutputPortMap=o1
  Sum1 : Sum  Inputs=|++
  Sum2 : Sum  Inputs=|++
  Timed to Event Signal : TimedToEventSignal
  TravelTime : Constant  Value=35.7125/30
  IN_Shipment_1 : PMIOPort  Port=1  Side=Left
  OUT_Shipment_1 : PMIOPort  Port=2  Side=Right
  IN_Resource_1 : PMIOPort  Port=3  Side=Left
  OUT_Resource_1 : PMIOPort  Port=4  Side=Right
  IN_Shipment_2 : PMIOPort  Port=5  Side=Left
  OUT_Shipment_2 : PMIOPort  Port=6  Side=Right
  IN_Resource_2 : PMIOPort  Port=7  Side=Left
  OUT_Resource_2 : PMIOPort  Port=8  Side=Right
  wires:
  Inbound_Release_2/1 -> Sum2/2
  Outbound_Release_1/1 -> Sum2/1
  Sum2/1 -> Enabled Gate/1
  Inbound_Release_1/1 -> Sum1/1
  Outbound_Release_2/1 -> Sum1/2
  Sum1/1 -> Enabled Gate1/1
  Timed to Event Signal/1 -> Outbound_Process_2/1, Outbound_Process_1/1, Infinite Server1/1, Inbound_Process_2/1, Inbound_Process_1/1, Infinite Server/1
  TravelTime/1 -> Timed to Event Signal/1
  connections:
  Inbound_Process_1/RConn1 -- OUT_Resource_1/RConn1
  Outbound_Process_1/RConn1 -- Inbound_Release_1/LConn1
  Inbound_Release_1/RConn1 -- Inbound_Process_1/LConn1
  Outbound_Release_1/RConn1 -- Outbound_Process_1/LConn1
  Inbound_Process_2/RConn1 -- OUT_Resource_2/RConn1
  Inbound_Release_2/RConn1 -- Inbound_Process_2/LConn1
  Outbound_Process_2/RConn1 -- Inbound_Release_2/LConn1
  Outbound_Release_2/RConn1 -- Outbound_Process_2/LConn1
  IN_Resource_2/RConn1 -- Outbound_Release_2/LConn1
  Infinite Server1/RConn1 -- OUT_Shipment_1/RConn1
  Enabled Gate/RConn1 -- Infinite Server1/LConn1
  Infinite Server/LConn1 -- Enabled Gate1/RConn1
  OUT_Shipment_2/RConn1 -- Infinite Server/RConn1
  IN_Resource_1/RConn1 -- Outbound_Release_1/LConn1
  IN_Shipment_2/RConn1 -- FIFO Queue1/LConn1
  IN_Shipment_1/RConn1 -- FIFO Queue/LConn1
  Enabled Gate1/LConn1 -- FIFO Queue1/RConn1
  FIFO Queue/RConn1 -- Enabled Gate/LConn1
